simulink model "scd3busMicrogridDroopControlFidelityLevels3Inv"  (R2025b)
settings: Solver=ode15s  StartTime=0.0  StopTime=24  RelTol=1e-3
PreLoadFcn:
  | scd3busMicrogridDroopControlDataFidelityLevels3Inv;
  | 
  | %% Controller variants
  | % Create variant controls for converter controller. Controller has two
  | % different levels of fidelity: Averaged, AveragedPulse, Pulse
  | Averaged = Simulink.VariantExpression;
  | Averaged.Condition = 'fidelity==scd3busMicrogridDroopControl_variants_enum.Low';
  | Pulse = Simulink.VariantExpression;
  | Pulse.Condition = 'fidelity==scd3busMicrogridDroopControl_variants_enum.High';
  | 
  | %% Plant variants
  | % Create variant controls for converter plant. Plant has three different
  | % levels of fidelity.
  | AveragedNonSwitch = Simulink.VariantExpression;
  | AveragedNonSwitch.Condition = 'fidelity==scd3busMicrogridDroopControl_variants_enum.Low';
  | PulseSwitch = Simulink.VariantExpression;
  | PulseSwitch.Condition = 'fidelity==scd3busMicrogridDroopControl_variants_enum.High';
  | 
  | %% Set up variables ready for simulation
  | fidelity = scd3busMicrogridDroopControl_variants_enum.High;
  | Ts = 5e-6;
  | Ts_V = 1e-6;
  | Tsc = 1e-4;
  | Tsc_V = 5e-4;
values from neighbouring files (symbols this model uses):
  consensus_enable = 1    [scd3busMicrogridDroopControlDataFidelityLevels3Inv.m]
  fgrid = 60    [scd3busMicrogridDroopControlDataFidelityLevels.m]    (also in scd3busMicrogridDroopControlDataFidelityLevels3Inv.m)
  Kdroop_fp1 = 0.03/2    (= 0.015)    [scd3busMicrogridDroopControlDataFidelityLevels3Inv.m]
  Kdroop_fp2 = 0.03/2    (= 0.015)    [scd3busMicrogridDroopControlDataFidelityLevels3Inv.m]
  Kdroop_vq1 = 0.05/2    (= 0.025)    [scd3busMicrogridDroopControlDataFidelityLevels3Inv.m]
  Kdroop_vq2 = 0.05/2    (= 0.025)    [scd3busMicrogridDroopControlDataFidelityLevels3Inv.m]
  Ki_vd = 850    [scd3busMicrogridDroopControlDataFidelityLevels.m]    (also in scd3busMicrogridDroopControlDataFidelityLevels3Inv.m)
  Ki_vq = 850    [scd3busMicrogridDroopControlDataFidelityLevels.m]    (also in scd3busMicrogridDroopControlDataFidelityLevels3Inv.m)
  Kp_vd = 0.36    [scd3busMicrogridDroopControlDataFidelityLevels.m]    (also in scd3busMicrogridDroopControlDataFidelityLevels3Inv.m)
  Kp_vq = 0.36    [scd3busMicrogridDroopControlDataFidelityLevels.m]    (also in scd3busMicrogridDroopControlDataFidelityLevels3Inv.m)
  Vdc1 = 1000    [scd3busMicrogridDroopControlDataFidelityLevels.m]    (also in scd3busMicrogridDroopControlDataFidelityLevels3Inv.m)
  Vdc2 = 1000    [scd3busMicrogridDroopControlDataFidelityLevels.m]    (also in scd3busMicrogridDroopControlDataFidelityLevels3Inv.m)
  Vrms = 380    [scd3busMicrogridDroopControlDataFidelityLevels.m]    (also in scd3busMicrogridDroopControlDataFidelityLevels3Inv.m)
undefined symbols (not defined in the file or in its folder): DiscIntNeverNeededParam
libraries: ee_lib x29, nesl_utility x27, fl_lib x15, eeTransforms x4, eeSinusoidalMeasurement x4, slpidlib x4, eePwmGeneratorTwoLevel x2, eePowerMeasurement x2, simulink x2, SignalEditorBlockLib x1
(part 3 of 3)

== system scd3busMicrogridDroopControlFidelityLevels3Inv/Inverter 2/Solar2/MPPT Algorithm ==
  I : Inport
  V : Inport  Port=2
  D_init : Constant  Value=0.25
  D_max : Constant  Value=0.4
  D_min : Constant  Value=0.1
  Delta_D : Constant  Value=0.001
  MPPT Algorithm : MATLAB Function  SystemSampleTime=Ts
  Unit Delay : UnitDelay  InitialCondition=0.2  SampleTime=0.01
  Vector Concatenate : Concatenate  NumInputs=4
  duty_cycle : Outport
  wires:
  V/1 -> MPPT Algorithm/2(V)
  Vector Concatenate/1 -> MPPT Algorithm/1(Param)
  D_max/1 -> Vector Concatenate/2
  D_init/1 -> Vector Concatenate/1
  D_min/1 -> Vector Concatenate/3
  MPPT Algorithm/1(D) -> Unit Delay/1
  Delta_D/1 -> Vector Concatenate/4
  I/1 -> MPPT Algorithm/3(I)
  Unit Delay/1 -> duty_cycle/1

== system scd3busMicrogridDroopControlFidelityLevels3Inv/Inverter 2/Solar2/Sensing Current ==
  Current Sensor : fl_lib/Electrical/Electrical Sensors/Current Sensor
  PS-Simulink/I : nesl_utility/PS-Simulink Converter  PhysicalDomain=network_engine_domain  SubClassName=ps_output  LeftPortType=input  RightPortType=output  PseudoPeriodic=off  Frequencies=[]  VectorFormat=1-D array  Unit=1  AffineConversion=off
  + : PMIOPort  Side=Left
  - : PMIOPort  Port=2  Side=Right
  I : Outport
  wires:
  PS-Simulink/I/1 -> I/1
  connections:
  -/RConn1 -- Current Sensor/RConn2
  Current Sensor/LConn1 -- +/RConn1
  Current Sensor/RConn1 -- PS-Simulink/I/LConn1

== system scd3busMicrogridDroopControlFidelityLevels3Inv/Inverter 2/Solar2/sensing voltage ==
  PS-Simulink Converter : nesl_utility/PS-Simulink Converter  PhysicalDomain=network_engine_domain  SubClassName=ps_output  LeftPortType=input  RightPortType=output  PseudoPeriodic=off  Frequencies=[]  VectorFormat=1-D array  Unit=inherit  AffineConversion=off
  Voltage Sensor : fl_lib/Electrical/Electrical Sensors/Voltage Sensor
  + : PMIOPort  Side=Left
  - : PMIOPort  Port=2  Side=Right
  V : Outport
  wires:
  PS-Simulink Converter/1 -> V/1
  connections:
  Voltage Sensor/LConn1 -- +/RConn1
  Voltage Sensor/RConn2 -- -/RConn1
  Voltage Sensor/RConn1 -- PS-Simulink Converter/LConn1

== matlab function scd3busMicrogridDroopControlFidelityLevels3Inv/Inverter 2/Solar2/MPPT Algorithm/MPPT Algorithm ==
  settings: updateMethod=DISCRETE  sampleTime=Ts_DC
  data: Param input; V input; I input; D output
function D = PandO(Param, V, I)

Dinit  = Param(1);
Dmax   = Param(2);
Dmin   = Param(3);
deltaD = Param(4);

persistent Vold Pold Dold;
if isempty(Vold)
    Vold = 0;
    Pold = 0;
    Dold = Dinit;
end

P  = V * I;
dV = V - Vold;
dP = P - Pold;

%% -- fixed: use a dead-band instead of exact zero comparison --
if abs(dP) < 0.5        % ignore changes smaller than 0.5 W (noise)
    D = Dold;           % already at MPP, hold duty cycle

elseif dP < 0
    if dV < 0
        D = Dold - deltaD;
    else
        D = Dold + deltaD;
    end

else                    % dP > 0
    if dV < 0
        D = Dold + deltaD;
    else
        D = Dold - deltaD;
    end
end

%% -- clamp --
D = max(Dmin, min(Dmax, D));

%% -- update persistent state --
Dold = D;
Vold = V;
Pold = P;

== matlab function scd3busMicrogridDroopControlFidelityLevels3Inv/Inverter 1/Droop Controller Inverter1/MATLAB Function ==
  data: omega_1 input; d_omega output; omega_2 input; V_1 input; V_2 input; int_w_in input; int_v_in input; Ts input; d_V output; int_w_out output; int_v_out output
function [d_omega, d_V, int_w_out, int_v_out] = ...
         Consensus_Agent1(omega_1, omega_2, V_1, V_2, ...
                          int_w_in, int_v_in, Ts)
%% Gains — tuned for Hz units and visible correction
alpha_w = 100.0;   beta_w = 60.0;   kref_w = 40.0;
alpha_v = 0.60;   beta_v = 0.40;   kref_v = 0.20;

omega_ref = 60.0;   % Hz — confirmed from your freq_mea display
V_ref     = 1.0;    % pu

%% Frequency
e_omega     = omega_1 - omega_ref;
consensus_w = omega_1 - omega_2;
int_w_out   = max(-1, min(1, int_w_in + Ts * consensus_w));
d_omega     = -alpha_w*consensus_w - beta_w*int_w_out - kref_w*e_omega;
d_omega     = max(-4.0, min(4.0, d_omega));   % wider clamp

%% Voltage
e_V         = V_1 - V_ref;
consensus_v = V_1 - V_2;
int_v_out   = max(-0.40, min(0.40, int_v_in + Ts * consensus_v));
d_V         = -alpha_v*consensus_v - beta_v*int_v_out - kref_v*e_V;
d_V         = max(-0.30, min(0.30, d_V));
end

== matlab function scd3busMicrogridDroopControlFidelityLevels3Inv/Inverter 2/Droop Controller Inverter2/MATLAB Function ==
  data: omega_2 input; d_omega output; omega_1 input; V_2 input; V_1 input; int_w_in input; int_v_in input; Ts input; d_V output; int_w_out output; int_v_out output
function [d_omega, d_V, int_w_out, int_v_out] = ...
         Consensus_Agent2(omega_2, omega_1, V_2, V_1, ...
                          int_w_in, int_v_in, Ts)
%% Identical gains to Agent 1
alpha_w = 100.0;   beta_w = 60.0;   kref_w = 40.0;
alpha_v = 0.60;   beta_v = 0.40;   kref_v = 0.20;

omega_ref = 60.0;
V_ref     = 1.0;

%% Frequency
e_omega     = omega_2 - omega_ref;
consensus_w = omega_2 - omega_1;
int_w_out   = max(-1, min(1, int_w_in + Ts * consensus_w));
d_omega     = -alpha_w*consensus_w - beta_w*int_w_out - kref_w*e_omega;
d_omega     = max(-4.0, min(4.0, d_omega));

%% Voltage
e_V         = V_2 - V_ref;
consensus_v = V_2 - V_1;
int_v_out   = max(-0.40, min(0.40, int_v_in + Ts * consensus_v));
d_V         = -alpha_v*consensus_v - beta_v*int_v_out - kref_v*e_V;
d_V         = max(-0.30, min(0.30, d_V));
end

== matlab function scd3busMicrogridDroopControlFidelityLevels3Inv/Inverter 1/Solar1/MPPT Algorithm/MPPT Algorithm ==
  settings: updateMethod=DISCRETE  sampleTime=Ts_DC
  data: Param input; V input; I input; D output
function D = PandO(Param, V, I)

Dinit  = Param(1);
Dmax   = Param(2);
Dmin   = Param(3);
deltaD = Param(4);

persistent Vold Pold Dold;
if isempty(Vold)
    Vold = 0;
    Pold = 0;
    Dold = Dinit;
end

P  = V * I;
dV = V - Vold;
dP = P - Pold;

%% -- fixed: use a dead-band instead of exact zero comparison --
if abs(dP) < 0.5        % ignore changes smaller than 0.5 W (noise)
    D = Dold;           % already at MPP, hold duty cycle

elseif dP < 0
    if dV < 0
        D = Dold - deltaD;
    else
        D = Dold + deltaD;
    end

else                    % dP > 0
    if dV < 0
        D = Dold + deltaD;
    else
        D = Dold - deltaD;
    end
end

%% -- clamp --
D = max(Dmin, min(Dmax, D));

%% -- update persistent state --
Dold = D;
Vold = V;
Pold = P;
